simulink model "try_2"  (R2021b)
settings: Solver=VariableStepAuto  StartTime=0.0  StopTime=10  RelTol=1e-3
libraries: roblocks x1
settings Model: Creator=Administrator  LastModifiedBy=Administrator

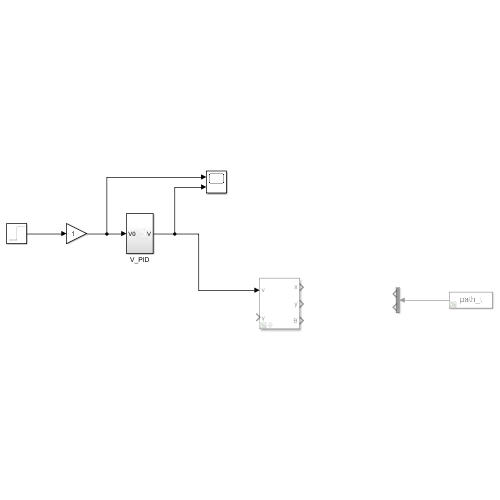
[thumbnail: Simulink's stored preview of the top-level diagram]
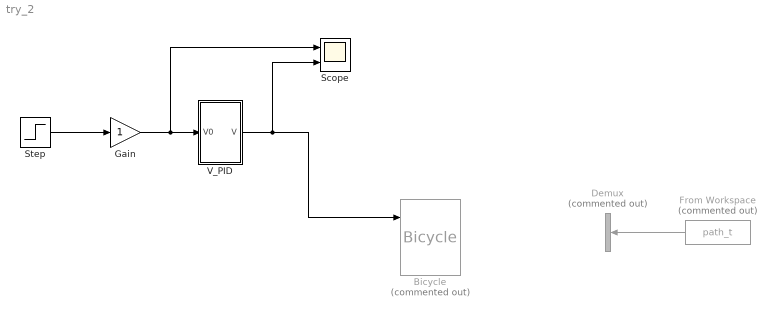
== system try_2 ==
  Bicycle : roblocks/Vehicles/Bicycle  Commented=on  vlim=1  accel=Inf  alim=2  steer_rate=Inf  L=1  x0=[0, 0, 0]
  Demux : Demux  Commented=on  Outputs=2
  From Workspace : FromWorkspace  Commented=on  VariableName=path_t
  Gain : Gain
  Scope : Scope  NumInputPorts=2
  Step : Step  Time=0  SampleTime=0
  V_PID : Subsystem
  wires:
  V_PID/1(V) -> Scope/2, Bicycle/1
  From Workspace/1 -> Demux/1
  Step/1 -> Gain/1
  Gain/1 -> Scope/1, V_PID/1(V0)

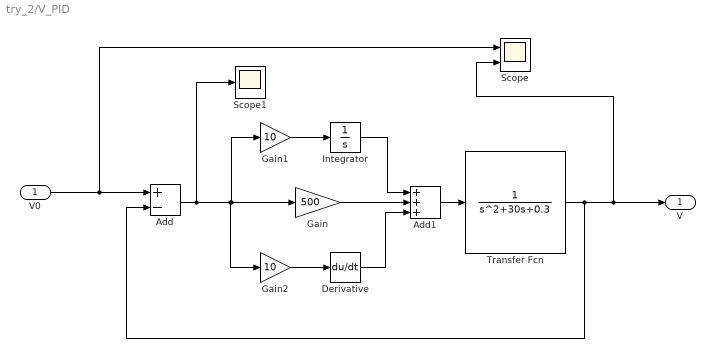
== system try_2/V_PID ==
  V0 : Inport
  Add : Sum  Inputs=+-
  Add1 : Sum  Inputs=+++
  Derivative : Derivative
  Gain : Gain  Gain=500
  Gain1 : Gain  Gain=10
  Gain2 : Gain  Gain=10
  Integrator : Integrator
  Scope : Scope  NumInputPorts=2
  Scope1 : Scope
  Transfer Fcn : TransferFcn  Denominator=[1 30 0.3]
  V : Outport
  wires:
  V0/1 -> Scope/1, Add/1
  Add1/1 -> Transfer Fcn/1
  Add/1 -> Scope1/1, Gain2/1, Gain1/1, Gain/1
  Gain1/1 -> Integrator/1
  Transfer Fcn/1 -> Add/2, Scope/2, V/1
  Derivative/1 -> Add1/3
  Integrator/1 -> Add1/1
  Gain/1 -> Add1/2
  Gain2/1 -> Derivative/1
